simulink model "verify_sfunBoiler_mdl"  (R2016b)
settings: Solver=ode45  StartTime=0.0  StopTime=3600  MaxStep=300  RelTol=1e-3  EnableMultiTasking=on
libraries: carnot x2
settings Model: Creator=drhf  LastModifiedBy=drhf
settings DataIOCC: LimitDataPoints=on  SaveFormat=Array  SignalLoggingSaveFormat=ModelDataLogs
settings OptimizationCC: ExpressionDepthLimit=2147483647  LifeSpan=inf
settings DebuggingCC: UnderspecifiedInitializationDetection=Classic  MergeDetectMultiDrivingBlocksExec=none  SolverPrmCheckMsg=warning  FcnCallInpInsideContextMsg=warning  StateNameClashWarn=warning  SFUnexpectedBacktrackingDiag=warning  SFNoUnconditionalDefaultTransitionDiag=warning  SFExecutionAtInitializationDiag=none
settings HardwareCC: ProdBitPerPointer=32  ProdBitPerSizeT=32  ProdBitPerPtrDiffT=32  ProdLargestAtomicFloat=None  ProdIntDivRoundTo=Undefined  ProdEndianess=Unspecified  ProdWordSize=32  ProdHWDeviceType=32-bit Generic
settings ModelReferenceCC: PropagateSignalLabelsOutOfModel=off
settings GRTTargetCC: TargetLangStandard=C89/C90 (ANSI)  GeneratePreprocessorConditionals=Disable all  CombineOutputUpdateFcns=off  GRTInterface=on
settings ConfigComp: CovMetricSettings=dw  CovHtmlReporting=on  CovSaveCumulativeToWorkspaceVar=on  CovSaveSingleToWorkspaceVar=on  CovExternalEMLEnable=off

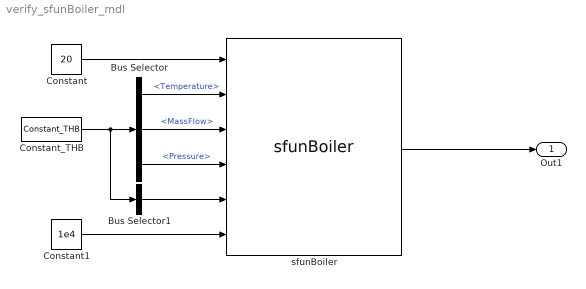
== system verify_sfunBoiler_mdl ==
  Bus Selector : BusSelector  OutputSignals=Temperature,MassFlow,Pressure
  Bus Selector1 : BusSelector  OutputSignals=FluidType,FluidMix  OutputAsBus=on
  Constant : Constant  Value=20
  Constant1 : Constant  Value=1e4
  Constant_THB : carnot/Source/Simple/Constant_THB  t=30  mdot=1e4/4182/20  p=2e5  mID=No Pressure Drop  fluid=Water  mix=0  mix2=0  mix3=0  dia=0.02  hgt=0
  sfunBoiler : carnot/Basic/Thermal_Models/sfunBoiler  UA=1  vol=0.01  Tini=50  nodes=1
  Out1 : Outport
  wires:
  Constant/1 -> sfunBoiler/1
  sfunBoiler/1 -> Out1/1
  Constant1/1 -> sfunBoiler/6
  Constant_THB/1 -> Bus Selector1/1, Bus Selector/1
  Bus Selector/3 -> sfunBoiler/4  "<Pressure>"
  Bus Selector/2 -> sfunBoiler/3  "<MassFlow>"
  Bus Selector/1 -> sfunBoiler/2  "<Temperature>"
  Bus Selector1/1 -> sfunBoiler/5
